simulink model "base4"  (R2023b)
settings: Solver=VariableStepAuto  StartTime=0.0  StopTime=100  RelTol=1e-3
settings Model: Creator=21917  LastModifiedBy=21917

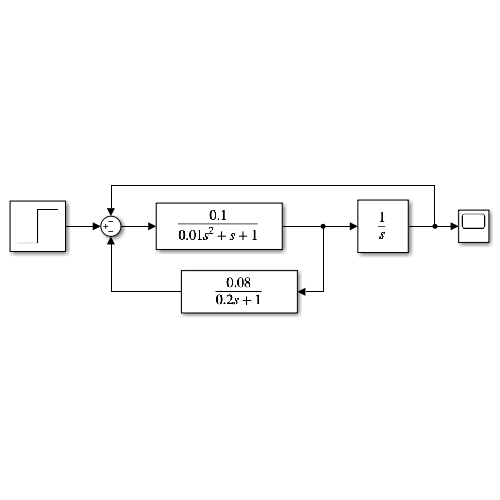
[thumbnail: Simulink's stored preview of the top-level diagram]
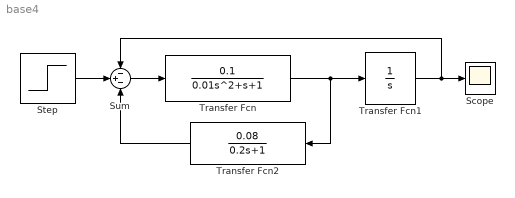
== system base4 ==
  Scope : Scope
  Step : Step  SampleTime=0
  Sum : Sum  Inputs=-+-
  Transfer Fcn : TransferFcn  Numerator=[0.1]  Denominator=[0.01 1 1]
  Transfer Fcn1 : TransferFcn  Denominator=[1 0]
  Transfer Fcn2 : TransferFcn  Numerator=[0.08]  Denominator=[0.2 1]
  wires:
  Transfer Fcn/1 -> Transfer Fcn1/1, Transfer Fcn2/1
  Sum/1 -> Transfer Fcn/1
  Transfer Fcn1/1 -> Scope/1, Sum/1
  Step/1 -> Sum/2
  Transfer Fcn2/1 -> Sum/3
